simulink model "Blockdiagram"  (R2018a)
settings: Solver=VariableStepAuto  StartTime=0.0  StopTime=10.0  RelTol=1e-3
settings Model: Creator=mairo  LastModifiedBy=mairo

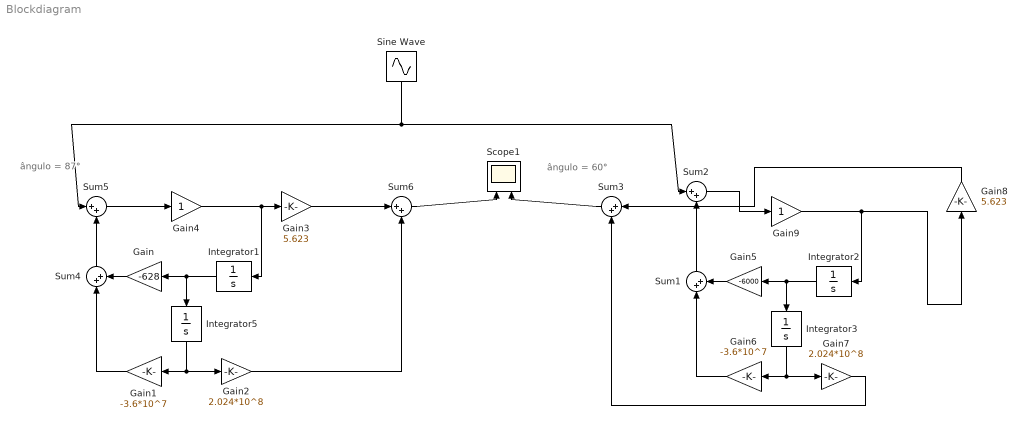
== system Blockdiagram ==
  note: ângulo = 60°
  note: ângulo = 87°
  Gain : Gain  Gain=-628
  Gain1 : Gain  Gain=-3.6*10^7
  Gain2 : Gain  Gain=2.024*10^8
  Gain3 : Gain  Gain=5.623
  Gain4 : Gain
  Gain5 : Gain  Gain=-6000
  Gain6 : Gain  Gain=-3.6*10^7
  Gain7 : Gain  Gain=2.024*10^8
  Gain8 : Gain  Gain=5.623
  Gain9 : Gain
  Integrator{1..3,5} (4 alike) : Integrator
  Scope1 : Scope  NumInputPorts=2
  Sine Wave : Sin  Amplitude=10  Frequency=6000  SampleTime=0
  Sum{1..6} (6 alike) : Sum  Inputs=|++
  wires:
  Gain4/1 -> Gain3/1, Integrator1/1
  Integrator1/1 -> Gain/1, Integrator5/1
  Gain/1 -> Sum4/2
  Integrator5/1 -> Gain2/1, Gain1/1
  Gain1/1 -> Sum4/1
  Sum5/1 -> Gain4/1
  Sum4/1 -> Sum5/2
  Gain2/1 -> Sum6/2
  Gain3/1 -> Sum6/1
  Gain8/1 -> Sum3/1
  Sum1/1 -> Sum2/2
  Integrator3/1 -> Gain7/1, Gain6/1
  Gain7/1 -> Sum3/2
  Integrator2/1 -> Gain5/1, Integrator3/1
  Gain5/1 -> Sum1/2
  Sum2/1 -> Gain9/1
  Gain6/1 -> Sum1/1
  Gain9/1 -> Gain8/1, Integrator2/1
  Sum6/1 -> Scope1/1
  Sine Wave/1 -> Sum2/1, Sum5/1
  Sum3/1 -> Scope1/2
